simulink model "test_priklad1"  (R2017b)
settings: Solver=VariableStepAuto  StartTime=0.0  StopTime=10.0  RelTol=1e-3
libraries: simulink x1
settings Model: Creator=nanom  LastModifiedBy=nanom

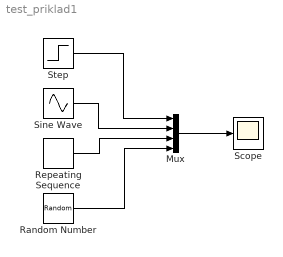
== system test_priklad1 ==
  Mux : Mux
  Random Number : RandomNumber  SampleTime=0.1
  Repeating Sequence : simulink/Sources/Repeating Sequence  rep_seq_t=[0 2]  rep_seq_y=[0 2]
  Scope : Scope
  Sine Wave : Sin  Amplitude=7  Frequency=3.14  Phase=1.5  SampleTime=0
  Step : Step  Time=2.5  Before=0.75  After=6  SampleTime=0
  wires:
  Mux/1 -> Scope/1
  Step/1 -> Mux/1
  Sine Wave/1 -> Mux/2
  Repeating Sequence/1 -> Mux/3
  Random Number/1 -> Mux/4
